simulink model "alphabetaPLL"  (R2020b)
settings: Solver=FixedStepAuto  StartTime=0.0  StopTime=36.72  FixedStep=1e-4  MaxStep=1e-4  MinStep=1e-6  RelTol=1e-3
undefined symbols (not defined in the file or in its folder): A_frq_step, A_phase_step, f_rad, t_frq_step, t_phase_step, V_g, var_noise
libraries: simulink x6, bach_library x2
settings Model: Creator=martin  LastModifiedBy=Kasper Laustsen
settings DataIOCC: ExternalInput=tt1, tt2, tt3, tt4, tt5, tt6  LoadExternalInput=on

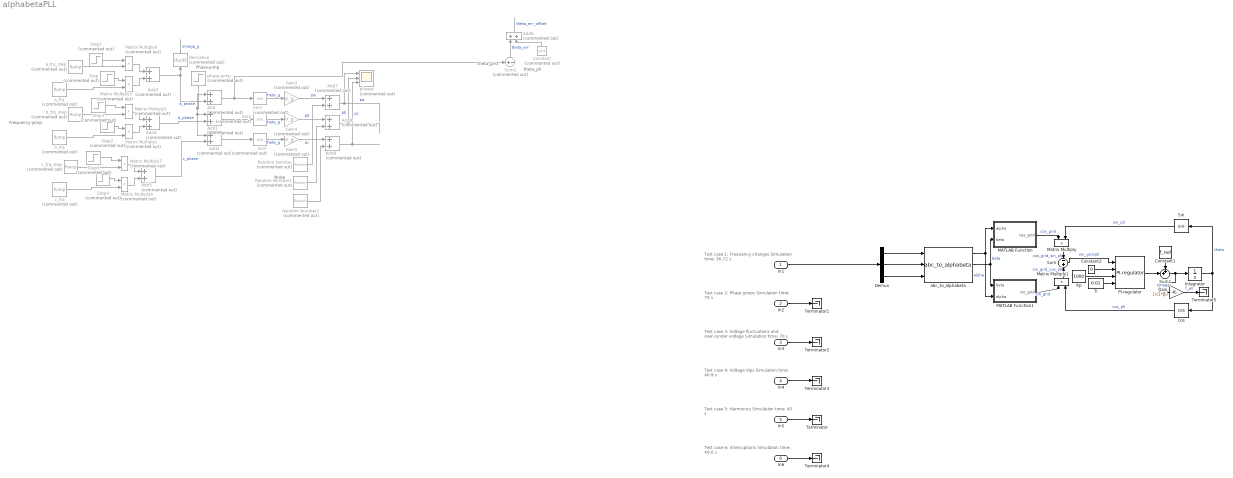
== system alphabetaPLL ==
  note: Noise
  note: theta_pll
  note: theta_grid
  note: Frequency-jump
  note: Phase-jump
  note: Test case 2: Phase jumps
      | Simulation time: 70 s
  note: Test case 1: Frequency changes
      | Simulation time: 36.72 s
  note: Test case 3: Voltage fluctuations
      | and over-/under voltage
      | Simulation time: 70 s
  note: Test case 4: Voltage dips
      | Simulation time: 40.9 s
  note: Test case 5: Harmonics
      | Simulation time: 40 s
  note: Test case 6: Interruptions
      | Simulation time: 40.6 s
  In1 : Inport  PortDimensions=3
  In2 : Inport  Port=2  PortDimensions=3
  In3 : Inport  Port=3  PortDimensions=3
  In4 : Inport  Port=4  PortDimensions=3
  In5 : Inport  Port=5  PortDimensions=3
  In6 : Inport  Port=6  PortDimensions=3
  Add{,1..9} (10 alike) : Sum  Commented=on
  Constant : Constant  Commented=on  Value=-pi/2
  Constant1 : Constant  Value=f_rad
  Constant2 : Constant  Value=0
  Cos : Trigonometry  Operator=cos
  Demux : Demux  Outputs=3
  Derivative : Derivative  Commented=on
  Gain : Gain  Gain=1/(2*pi)
  Gain3 : Gain  Commented=on  Gain=V_g
  Gain4 : Gain  Commented=on  Gain=V_g
  Gain5 : Gain  Commented=on  Gain=V_g
  Integrator : Integrator
  Kp : Constant  Value=1000
  MATLAB Function : MATLAB Function  TreatAsAtomicUnit=on
  MATLAB Function1 : MATLAB Function  TreatAsAtomicUnit=on
  Matrix Multiply : Product
  Matrix Multiply1 : Product
  Matrix Multiply{2..7} (6 alike) : Product  Commented=on
  PI-regulator : bach_library/PI-regulator  SystemSampleTime=-1  VariantActivationTime=update diagram  Latency=0  AutoFrameSizeCalculation=off
  Random Number : RandomNumber  Commented=on  Variance=var_noise
  Random Number1 : RandomNumber  Commented=on  Variance=var_noise  Seed=1
  Random Number2 : RandomNumber  Commented=on  Variance=var_noise  Seed=2
  Sin : Trigonometry
  Sin3 : Trigonometry  Commented=on
  Sin4 : Trigonometry  Commented=on
  Sin5 : Trigonometry  Commented=on
  Step : Step  Commented=on  Time=t_frq_step  Before=1  After=0  SampleTime=0
  Step1 : Step  Commented=on  Time=t_frq_step  SampleTime=0
  Step2 : Step  Commented=on  Time=t_frq_step  Before=1  After=0  SampleTime=0
  Step3 : Step  Commented=on  Time=t_frq_step  SampleTime=0
  Step4 : Step  Commented=on  Time=t_frq_step  Before=1  After=0  SampleTime=0
  Step5 : Step  Commented=on  Time=t_frq_step  SampleTime=0
  Sum : Sum  Inputs=-|+
  Sum1 : Sum  Inputs=++|
  Sum2 : Sum  Commented=on  Inputs=+|-
  Terminator{,1..5} (6 alike) : Terminator
  Ti : Constant  Value=0.01
  a_frq : simulink/Sources/Ramp  Commented=on  slope=f_rad  start=0  InitialOutput=0
  a_frq_step : simulink/Sources/Ramp  Commented=on  slope=f_rad*A_frq_step  start=t_frq_step  InitialOutput=t_frq_step*f_rad
  abc_to_alphabeta : bach_library/abc_to_alphabeta  SystemSampleTime=-1  VariantActivationTime=update diagram  Latency=0  AutoFrameSizeCalculation=off
  b_frq : simulink/Sources/Ramp  Commented=on  slope=f_rad  start=0  InitialOutput=f_rad/3
  b_frq_step : simulink/Sources/Ramp  Commented=on  slope=f_rad*A_frq_step  start=t_frq_step  InitialOutput=t_frq_step*f_rad+f_rad/3
  c_frq : simulink/Sources/Ramp  Commented=on  slope=f_rad  start=0  InitialOutput=f_rad*2/3
  c_frq_step : simulink/Sources/Ramp  Commented=on  slope=f_rad*A_frq_step  start=t_frq_step  InitialOutput=t_frq_step*f_rad+f_rad*2/3
  phase-jump : Step  Commented=on  Time=t_phase_step  After=A_phase_step  SampleTime=0
  phases : Scope  Commented=on  NumInputPorts=3
  wires:
  abc_to_alphabeta/1 -> MATLAB Function/1(alpha), MATLAB Function1/2(alpha)  "alpha"
  abc_to_alphabeta/2 -> MATLAB Function/2(beta), MATLAB Function1/1(beta)  "beta"
  Matrix Multiply1/1 -> Sum/2  "sin_grid_cos_pll"
  Matrix Multiply/1 -> Sum/1  "cos_grid_sin_pll"
  Ti/1 -> PI-regulator/4
  Kp/1 -> PI-regulator/3
  Sum/1 -> PI-regulator/1  "sin_grid-pll"
  Constant2/1 -> PI-regulator/2
  PI-regulator/1 -> Sum1/2
  Constant1/1 -> Sum1/1
  Add7/1 -> phases/1  "pa"
  Add8/1 -> phases/2  "pb"
  Add9/1 -> phases/3  "pc"
  Sum1/1 -> Gain/1, Integrator/1  "omega"
  Sin/1 -> Matrix Multiply/2  "sin_pll"
  Integrator/1 -> Sin/1, Cos/1  "theta"
  Cos/1 -> Matrix Multiply1/2  "cos_pll"
  Add3/1 -> Add/2, Derivative/1  "a_phase"
  Add4/1 -> Add1/2  "b_phase"
  Add5/1 -> Add2/2  "c_phase"
  phase-jump/1 -> Add/1, Add2/1, Add1/1
  Add2/1 -> Sin5/1
  Add1/1 -> Sin4/1
  Add/1 -> Sum2/1, Sin3/1
  a_frq/1 -> Matrix Multiply5/2
  Matrix Multiply6/1 -> Add3/1
  a_frq_step/1 -> Matrix Multiply6/2
  Matrix Multiply5/1 -> Add3/2
  Step/1 -> Matrix Multiply5/1
  Step1/1 -> Matrix Multiply6/1
  Step3/1 -> Matrix Multiply3/1
  Step2/1 -> Matrix Multiply2/1
  b_frq_step/1 -> Matrix Multiply3/2
  Matrix Multiply3/1 -> Add4/1
  b_frq/1 -> Matrix Multiply2/2
  Matrix Multiply2/1 -> Add4/2
  Step4/1 -> Matrix Multiply4/1
  Matrix Multiply7/1 -> Add5/1
  Matrix Multiply4/1 -> Add5/2
  c_frq_step/1 -> Matrix Multiply7/2
  Step5/1 -> Matrix Multiply7/1
  c_frq/1 -> Matrix Multiply4/2
  Derivative/1 -> ?  "omega_g"
  MATLAB Function1/1(sin_grid) -> Matrix Multiply1/1  "sin_grid"
  MATLAB Function/1(cos_grid) -> Matrix Multiply/1  "cos_grid"
  Sum2/1 -> Add6/1  "theta_err"
  Constant/1 -> Add6/2
  Add6/1 -> ?  "theta_err_offset"
  Sin3/1 -> Gain3/1  "theta_g"
  Sin4/1 -> Gain4/1  "theta_g"
  Sin5/1 -> Gain5/1  "theta_g"
  Random Number/1 -> Add7/2
  Gain5/1 -> Add9/1  "pc"
  Gain3/1 -> Add7/1  "pa"
  Gain4/1 -> Add8/1  "pb"
  Random Number1/1 -> Add8/2
  Random Number2/1 -> Add9/2
  In1/1 -> Demux/1
  Demux/1 -> abc_to_alphabeta/1
  Demux/2 -> abc_to_alphabeta/2
  Demux/3 -> abc_to_alphabeta/3
  In2/1 -> Terminator1/1
  In3/1 -> Terminator2/1
  In4/1 -> Terminator3/1
  In5/1 -> Terminator/1
  In6/1 -> Terminator4/1
  Gain/1 -> Terminator5/1  "f_pll"

== matlab function alphabetaPLL/MATLAB Function ==
  data: alpha input; cos_grid output; beta input
function cos_grid = cos_grid(alpha, beta)

cos_grid = alpha/sqrt(alpha^2+beta^2);

== matlab function alphabetaPLL/MATLAB Function1 ==
  data: beta input; alpha input; sin_grid output
function sin_grid = sin_grid(beta, alpha)

sin_grid = beta/sqrt(alpha^2+beta^2);
